simulink model "ofdm_transmitter"  (Simulink 8.5)
settings: Solver=ode45  StartTime=0.0  StopTime=inf  RelTol=1e-3
libraries: dspxfrm3 x2
settings Model: Creator=C4Josh  LastModifiedBy=C4Josh
settings DataIOCC: SignalLoggingSaveFormat=Dataset
settings OptimizationCC: BlockReduction=off  ConditionallyExecuteInputs=off  InlineParams=on  ExpressionDepthLimit=128
settings DebuggingCC: AlgebraicLoopMsg=error  UnderspecifiedInitializationDetection=Simplified  MergeDetectMultiDrivingBlocksExec=error  FcnCallInpInsideContextMsg=EnableAllAsError  StateNameClashWarn=none
settings HardwareCC: ProdHWDeviceType=ASIC/FPGA->ASIC/FPGA  ProdEqTarget=off
settings GRTTargetCC: CombineOutputUpdateFcns=on  GRTInterface=off
settings hdlcc: HDLCActiveTab=3

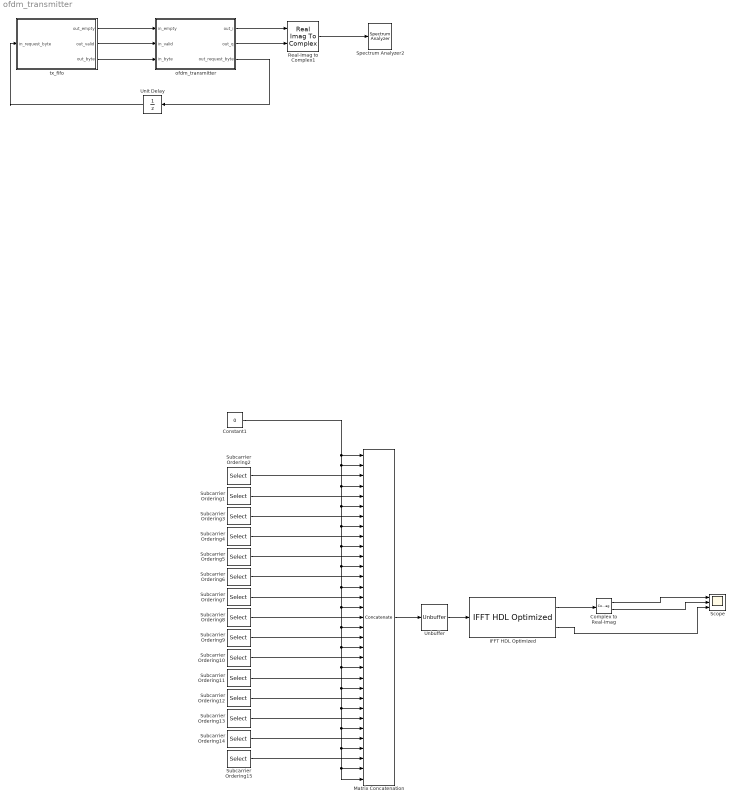
== system ofdm_transmitter ==
  Complex to Real-Imag : ComplexToRealImag
  Constant1 : Constant  Value=0  OutDataTypeStr=fixdt(1,12,7)
  IFFT HDL Optimized : dspxfrm3/IFFT HDL Optimized  BitReversedOutput=off  Normalize=on  FFTLengthSource=Property  FFTLength=64  RoundingMethod=Floor  OverflowAction=Saturate  ValidInputPort=off  ResetInputPort=off  StartOutputPort=off  EndOutputPort=off  SimulateUsing=Code generation
  Matrix Concatenation : Concatenate  NumInputs=33  Mode=Multidimensional array
  Real-Imag to Complex1 : RealImagToComplex
  Scope : Scope  NumInputPorts=3
      settings: YMin=-0.75~-0.75~1  YMax=1.5~0.75~1  SaveName=ScopeData2
  Spectrum Analyzer2 : SpectrumAnalyzer
  Subcarrier Ordering1 : Selector  InputPortWidth=45  Indices=4:6
  Subcarrier Ordering10 : Selector  InputPortWidth=45  Indices=28:30
  Subcarrier Ordering11 : Selector  InputPortWidth=45  Indices=31:33
  Subcarrier Ordering12 : Selector  InputPortWidth=45  Indices=34:36
  Subcarrier Ordering13 : Selector  InputPortWidth=45  Indices=37:39
  Subcarrier Ordering14 : Selector  InputPortWidth=45  Indices=40:42
  Subcarrier Ordering15 : Selector  InputPortWidth=45  Indices=40:42
  Subcarrier Ordering2 : Selector  InputPortWidth=45  Indices=1:3
  Subcarrier Ordering3 : Selector  InputPortWidth=45  Indices=7:9
  Subcarrier Ordering4 : Selector  InputPortWidth=45  Indices=10:12
  Subcarrier Ordering5 : Selector  InputPortWidth=45  Indices=13:15
  Subcarrier Ordering6 : Selector  InputPortWidth=45  Indices=16:18
  Subcarrier Ordering7 : Selector  InputPortWidth=45  Indices=19:21
  Subcarrier Ordering8 : Selector  InputPortWidth=45  Indices=22:24
  Subcarrier Ordering9 : Selector  InputPortWidth=45  Indices=25:27
  Unbuffer : Unbuffer  SampleBasedProcessing=Same as frame based
  Unit Delay : UnitDelay  SampleTime=-1
  ofdm_transmitter : Subsystem  TreatAsAtomicUnit=on
  tx_fifo : MATLAB Function  TreatAsAtomicUnit=on  SystemSampleTime=1/20e6
  wires:
  Subcarrier Ordering4/1 -> Matrix Concatenation/9
  Subcarrier Ordering11/1 -> Matrix Concatenation/23
  Subcarrier Ordering10/1 -> Matrix Concatenation/21
  Subcarrier Ordering8/1 -> Matrix Concatenation/17
  Subcarrier Ordering7/1 -> Matrix Concatenation/15
  Subcarrier Ordering3/1 -> Matrix Concatenation/7
  Subcarrier Ordering5/1 -> Matrix Concatenation/11
  Subcarrier Ordering15/1 -> Matrix Concatenation/31
  Subcarrier Ordering13/1 -> Matrix Concatenation/27
  Subcarrier Ordering9/1 -> Matrix Concatenation/19
  Subcarrier Ordering6/1 -> Matrix Concatenation/13
  IFFT HDL Optimized/1 -> Complex to Real-Imag/1
  IFFT HDL Optimized/2 -> Scope/3
  Constant1/1 -> Matrix Concatenation/2, Matrix Concatenation/4, Matrix Concatenation/6, Matrix Concatenation/8, Matrix Concatenation/10, Matrix Concatenation/14, Matrix Concatenation/16, Matrix Concatenation/20, Matrix Concatenation/24, Matrix Concatenation/26, Matrix Concatenation/32, Matrix Concatenation/33, Matrix Concatenation/30, Matrix Concatenation/28, Matrix Concatenation/22, Matrix Concatenation/18, Matrix Concatenation/12, Matrix Concatenation/1
  Complex to Real-Imag/1 -> Scope/1
  Complex to Real-Imag/2 -> Scope/2
  Subcarrier Ordering1/1 -> Matrix Concatenation/5
  Subcarrier Ordering14/1 -> Matrix Concatenation/29
  Subcarrier Ordering12/1 -> Matrix Concatenation/25
  Matrix Concatenation/1 -> Unbuffer/1
  Unbuffer/1 -> IFFT HDL Optimized/1
  Subcarrier Ordering2/1 -> Matrix Concatenation/3
  Real-Imag to Complex1/1 -> Spectrum Analyzer2/1
  tx_fifo/1(out_empty) -> ofdm_transmitter/1(in_empty)
  tx_fifo/2(out_valid) -> ofdm_transmitter/2(in_valid)
  tx_fifo/3(out_byte) -> ofdm_transmitter/3(in_byte)
  ofdm_transmitter/1(out_i) -> Real-Imag to Complex1/1
  ofdm_transmitter/2(out_q) -> Real-Imag to Complex1/2
  ofdm_transmitter/3(out_request_byte) -> Unit Delay/1
  Unit Delay/1 -> tx_fifo/1(in_request_byte)

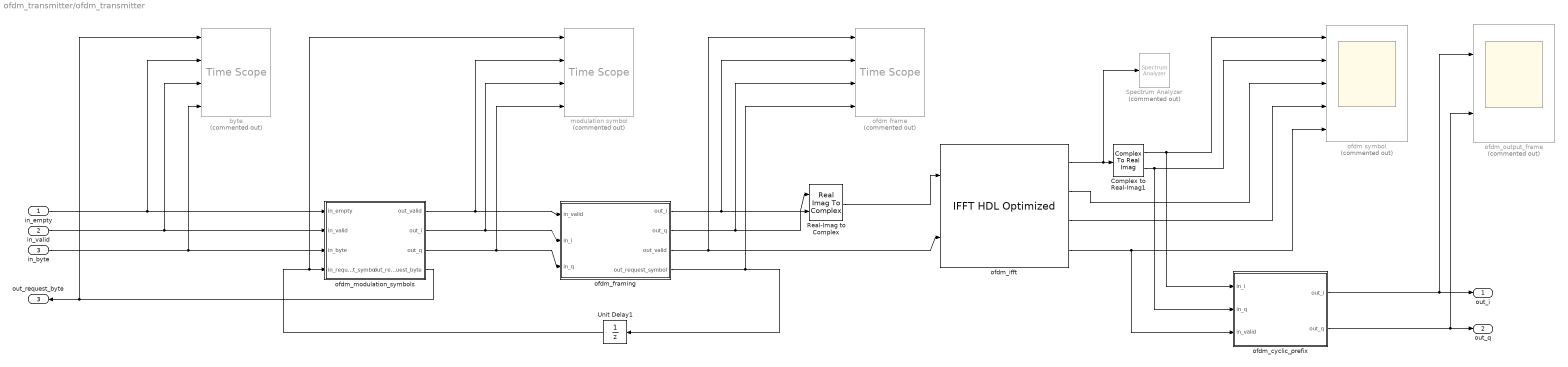
== system ofdm_transmitter/ofdm_transmitter ==
  in_empty : Inport
  in_valid : Inport  Port=2
  in_byte : Inport  Port=3
  " modulation symbol" : TimeScope  Commented=on  DefaultConfigurationName=spbscopes.TimeScopeBlockCfg  NumInputPorts=4
  Complex to Real-Imag1 : ComplexToRealImag
  Real-Imag to Complex : RealImagToComplex
  Spectrum Analyzer : SpectrumAnalyzer  Commented=on
  Unit Delay1 : UnitDelay  SampleTime=-1
  byte : TimeScope  Commented=on  DefaultConfigurationName=spbscopes.TimeScopeBlockCfg  NumInputPorts=4
  ofdm frame : TimeScope  Commented=on  DefaultConfigurationName=spbscopes.TimeScopeBlockCfg  NumInputPorts=4
  ofdm symbol : Scope  Commented=on  NumInputPorts=5
      settings: ShowLegends=on  YMin=-0.4~-0.75~0~0~0.95  YMax=0.4~0.75~1~1~1.05  SaveName=ScopeData3
  ofdm_cyclic_prefix : MATLAB Function  TreatAsAtomicUnit=on
  ofdm_framing : MATLAB Function  TreatAsAtomicUnit=on
  ofdm_ifft : dspxfrm3/IFFT HDL Optimized  BitReversedOutput=off  Normalize=on  FFTLengthSource=Property  FFTLength=64  RoundingMethod=Floor  OverflowAction=Saturate  ValidInputPort=on  ResetInputPort=off  StartOutputPort=on  EndOutputPort=on  SimulateUsing=Code generation
  ofdm_modulation_symbols : MATLAB Function  TreatAsAtomicUnit=on
  ofdm_output_frame : Scope  Commented=on  NumInputPorts=2
      settings: TickLabels=on  ShowLegends=on  TimeRange=800  YMin=-0.4~-0.7  YMax=0.35~0.7
  out_i : Outport
  out_q : Outport  Port=2
  out_request_byte : Outport  Port=3
  wires:
  in_empty/1 -> byte/2, ofdm_modulation_symbols/1(in_empty)
  in_valid/1 -> byte/3, ofdm_modulation_symbols/2(in_valid)
  in_byte/1 -> byte/4, ofdm_modulation_symbols/3(in_byte)
  ofdm_modulation_symbols/4(out_request_byte) -> out_request_byte/1, byte/1
  ofdm_modulation_symbols/1(out_valid) -> " modulation symbol"/2, ofdm_framing/1(in_valid)
  Unit Delay1/1 -> " modulation symbol"/1, ofdm_modulation_symbols/4(in_request_symbol)
  ofdm_modulation_symbols/2(out_i) -> " modulation symbol"/3, ofdm_framing/2(in_i)
  ofdm_modulation_symbols/3(out_q) -> " modulation symbol"/4, ofdm_framing/3(in_q)
  ofdm_framing/4(out_request_symbol) -> ofdm frame/4, Unit Delay1/1
  ofdm_framing/3(out_valid) -> ofdm frame/1, ofdm_ifft/2
  ofdm_framing/1(out_i) -> ofdm frame/2, Real-Imag to Complex/1
  ofdm_framing/2(out_q) -> ofdm frame/3, Real-Imag to Complex/2
  Real-Imag to Complex/1 -> ofdm_ifft/1
  ofdm_ifft/1 -> Complex to Real-Imag1/1, Spectrum Analyzer/1
  Complex to Real-Imag1/1 -> ofdm_cyclic_prefix/1(in_i), ofdm symbol/1
  Complex to Real-Imag1/2 -> ofdm_cyclic_prefix/2(in_q), ofdm symbol/2
  ofdm_ifft/2 -> ofdm symbol/3
  ofdm_ifft/3 -> ofdm symbol/4
  ofdm_ifft/4 -> ofdm_cyclic_prefix/3(in_valid), ofdm symbol/5
  ofdm_cyclic_prefix/2(out_q) -> ofdm_output_frame/2, out_q/1
  ofdm_cyclic_prefix/1(out_i) -> ofdm_output_frame/1, out_i/1

== matlab function ofdm_transmitter/ofdm_modulation_symbols ==
  data: out_valid output boolean size=1; out_i output fixdt(1,12,7) size=1; out_q output fixdt(1,12,7) size=1; in_empty input boolean size=1; in_valid input boolean size=1; out_request_byte output boolean size=1; in_byte input uint8 size=1; in_request_symbol input boolean size=1
function [out_valid, out_i, out_q, out_request_byte] = fcn(in_empty, in_valid, in_byte, in_request_symbol)
%#codegen

null = fi(0,1,12,7);

% MODULATION SYMBOL FORMAT
% 4-QAM, Grey coded, Minimum distance 2
%symbols = fi([-1+j -1-j 1+j 1-j],1,12,7);
symbols_i = fi([-1 -1 1 1],1,12,7);
symbols_q = fi([1 -1 1 -1],1,12,7);
bits_per_symbol = int8(2);
symbols_per_byte = 8/bits_per_symbol;
    
% by default, do nothing
out_request_byte = false;
out_i = null;
out_q = null;
out_valid = false;

% circular buffer for symbol storage
% the buffer length should evenly divide the number of symbols/byte
persistent buffer_i
if isempty(buffer_i)  
    buffer_i = repmat(null,1,2*symbols_per_byte);
end
persistent buffer_q
if isempty(buffer_q)  
    buffer_q = repmat(null,1,2*symbols_per_byte);
end
persistent read_index
if isempty(read_index)
    read_index = int8(0)
end
persistent write_index
if isempty(write_index)
    write_index = int8(0);
end

% we only receive valid input if we requested it
% if we have valid input, store the input
% this should *never* overflow
if in_valid
    
    % There are four symbols per byte
    % Map two bits to each symbol
    % This makes assumptions about the length of buffer
    % @review Is this the best way to do this?
    symbol1 = 1+bitand(bitshift(in_byte,-0),3);
    buffer_i(write_index+1) = symbols_i(symbol1);
    buffer_q(write_index+1) = symbols_q(symbol1);
    
    symbol2 = 1+bitand(bitshift(in_byte,-2),3);
    buffer_i(write_index+2) = symbols_i(symbol2);
    buffer_q(write_index+2) = symbols_q(symbol2);
    
    symbol3 = 1+bitand(bitshift(in_byte,-4),3);
    buffer_i(write_index+3) = symbols_i(symbol3);
    buffer_q(write_index+3) = symbols_q(symbol3);
    
    symbol4 = 1+bitand(bitshift(in_byte,-6),3);
    buffer_i(write_index+4) = symbols_i(symbol4);
    buffer_q(write_index+4) = symbols_q(symbol4);

    % we just wrote four symbols
    write_index = write_index + symbols_per_byte;
    if write_index >= length(buffer_i)
        write_index = int8(0);
    end
end

% determine how many symbols are buffered
buffered = int8(0);
if (read_index > write_index)
    buffered = (length(buffer_i) - read_index) + write_index;
elseif (read_index <= write_index)
    buffered = (write_index - read_index);
end

% if we have room for more symbols, request another byte
available = length(buffer_i) - buffered;
out_request_byte = (in_empty == 0) && (available >= symbols_per_byte);
%fprintf('[mod]read %d write %d request %d length %d buffered %d\n', ...
%    int8(read_index), int8(write_index), ...
%    int8(out_request_byte), int8(length(buffer_i)), int8(buffered));

% if there's buffered data, output a symbol
if in_request_symbol && (read_index ~= write_index)
    out_valid = true;
    out_i = buffer_i(read_index + 1);
    out_q = buffer_q(read_index + 1);
%    fprintf('[mod]read %d write %d symbol %d,%d\n', ...
%        int8(read_index), int8(write_index), ...
%        int8(out_i), int8(out_q));
    read_index = read_index + 1;
    if read_index >= length(buffer_i)
        read_index = int8(0);
    end
end

== matlab function tx_fifo ==
  data: out_empty output boolean size=1; out_valid output boolean size=1; in_request_byte input boolean size=1; out_byte output uint8 size=1
function [out_empty, out_valid, out_byte] = fcn(in_request_byte)
%#codegen

% assume we never empty
out_empty = false;

% we do not output by default
out_byte = uint8(0);
out_valid = false;

% fake data for our never empty source
persistent fake_data
if isempty(fake_data)
    fake_data = 3;
end

% if a byte is requested, supply a byte's worth of data
if in_request_byte
    out_byte = uint8(228);
    out_valid = true;
end

== matlab function ofdm_transmitter/ofdm_framing ==
  data: out_i output double; out_q output double; in_valid input double; in_i input double; in_q input double; out_valid output double; out_request_symbol output double
function [out_i, out_q, out_valid, out_request_symbol] = fcn(in_valid, in_i, in_q)
%#codegen

null = fi(0,1,12,7);
frame_size = int8(64);
% the number of symbols grouped in contiguous subcarries
symbols_per_run = 3;
% pilots are inserted between symbol runs
pilots_i = fi([1 0 -1 0],1,12,7);
pilots_q = fi([0 1 0 -1],1,12,7);

% this creates a frame that looks like:
% [ null null (pilot run)+ null ]
% given the current parameters, that means
% 16 pilots / ofdm frame
% 3xnull / ofdm frame
% 45 modulation symbols / ofdm frame
% 2 bits / modulation symbol
% 90 bits / ofdm frame

% default behavior
out_request_symbol = false;
out_valid = false;
out_i = null;
out_q = null;

% circular buffer for symbol storage
persistent buffer_i
if isempty(buffer_i)  
    buffer_i = repmat(null,1,frame_size);
end
persistent buffer_q
if isempty(buffer_q)  
    buffer_q = repmat(null,1,frame_size);
end
persistent read_index
if isempty(read_index)
    read_index = int8(0);
end
persistent write_index
if isempty(write_index)
    write_index = int8(0);
end

% framing state
persistent frame_index
persistent pilot_index
if isempty(pilot_index)
    pilot_index = int8(1);
end
persistent symbol_count
if isempty(symbol_count)
    symbol_count = int8(0);
end

% is this the first symbol in a frame?
frame_begin = (write_index == 0);
% is this the last symbol in a run?
run_end = (symbol_count == (symbols_per_run - 1));
% is this the last write in the frame?
% the frame will end with a (symbol)(pilot)(null)
frame_end = ((write_index + 2) == (frame_size - 1));
%fprintf('[frm]valid %d %f,%f write %d frame begin %d end %d run %d end %d\n', ...
%    int8(in_valid), double(in_i), double(in_q), ...
%    int8(write_index), ...
%    int8(frame_begin), int8(frame_end), ...
%    int8(symbol_count), int8(run_end));

% The following scenarios can occur:
% (null)(null)(pilot)(symbol)
% (symbol)(pilot)(null)
% (symbol)(pilot)
% (symbol)
if in_valid
    if frame_begin
        % (null)(null)(pilot)(symbol)
%        fprintf('[frm]write %d nullx2 pilot %d %d,%d symbol %d %d,%d\n', ...
%            int8(write_index), ...
%            int8(pilot_index), int8(pilots_i(pilot_index)), int8(pilots_q(pilot_index)), ...
%            int8(symbol_count), int8(in_i), int8(in_q));
        buffer_i(write_index+1) = null;
        buffer_q(write_index+1) = null;
        buffer_i(write_index+2) = null;
        buffer_q(write_index+2) = null;
        buffer_i(write_index+3) = pilots_i(1);
        buffer_q(write_index+3) = pilots_q(1);
        buffer_i(write_index+4) = in_i;
        buffer_q(write_index+4) = in_q;
        write_index = int8(4);
        symbol_count = int8(1);
        pilot_index = int8(2);
    elseif frame_end
        % (symbol)(pilot)(null)
%        fprintf('[frm]write %d symbol %d %d,%d pilot %d %d,%d null\n', ...
%            int8(write_index), ...
%            int8(symbol_count), int8(in_i), int8(in_q), ...
%            int8(pilot_index), int8(pilots_i(pilot_index)), int8(pilots_q(pilot_index)));
        buffer_i(write_index+1) = in_i;
        buffer_q(write_index+1) = in_q;
        buffer_i(write_index+2) = pilots_i(pilot_index);
        buffer_q(write_index+2) = pilots_q(pilot_index);
        buffer_i(write_index+3) = null;
        buffer_q(write_index+3) = null;
        write_index = int8(0);
        symbol_count = int8(0);
        pilot_index = int8(1);
    elseif run_end
        % (symbol)(pilot)
%        fprintf('[frm]write %d symbol %d %d,%d pilot %d %d,%d\n', ...
%            int8(write_index), ...
%            int8(symbol_count), int8(in_i), int8(in_q), ...
%            int8(pilot_index), int8(pilots_i(pilot_index)), int8(pilots_q(pilot_index)));
        buffer_i(write_index+1) = in_i;
        buffer_q(write_index+1) = in_q;
        buffer_i(write_index+2) = pilots_i(pilot_index);
        buffer_q(write_index+2) = pilots_q(pilot_index);
        write_index = write_index + 2;
        symbol_count = int8(0);
        pilot_index = pilot_index + 1;
        if pilot_index == length(pilots_i)
            pilot_index = int8(1);
        end
    else
        % (symbol)
%        fprintf('[frm]write %d symbol %d %d,%d\n', ...
%            int8(write_index), ...
%            int8(symbol_count), int8(in_i), int8(in_q));
        buffer_i(write_index+1) = in_i;
        buffer_q(write_index+1) = in_q;
        write_index = write_index + 1;
        symbol_count = symbol_count + 1;
    end
end

% determine how many symbols are buffered
buffered = int8(0);
if (read_index > write_index)
    buffered = (length(buffer_i) - read_index) + write_index;
elseif (read_index <= write_index)
    buffered = (write_index - read_index);
end

% we can write at *most* a 2xnull, a pilot, and a symbol
% if there's room enough to support as much, reques t a symbol
available = length(buffer_i) - buffered;
out_request_symbol = (available >= 4);

% output i/q if there's something buffered
if read_index ~= write_index
    out_valid = true;
    out_i = buffer_i(read_index + 1);
    out_q = buffer_q(read_index + 1);
    read_index = read_index + 1;
    if read_index >= length(buffer_i)
        read_index = int8(0);
    end
end

== matlab function ofdm_transmitter/ofdm_cyclic_prefix ==
  data: out_i output fixdt(1,12,7) size=1; out_q output fixdt(1,12,7) size=1; in_i input fixdt(1,12,7) size=1; in_q input fixdt(1,12,7) size=1; in_valid input boolean size=1
function [out_i, out_q]  = fcn(in_i, in_q, in_valid)
%#codegen

% constants
% ifft_size = 64;
% cyclic_prefix = 16;
null = fi(0,1,12,7);

% persistent state
persistent buffer_i
if isempty(buffer_i)  
    buffer_i = repmat(null,1,80);
end
persistent buffer_q
if isempty(buffer_q)  
    buffer_q = repmat(null,1,80);
end
persistent read_index
if isempty(read_index)
    read_index = int8(0);
end
persistent write_index
if isempty(write_index)
    write_index = int8(16);
end

% default behavior
out_i = null;
out_q = null;

% determine how many samples are buffered
buffered = int8(0);
if (read_index > write_index)
    buffered = (length(buffer_i) - read_index) + write_index;
elseif (read_index <= write_index)
    buffered = (write_index - read_index);
end

% if there's more than a cyclic prefix worth of space available,
% request input
available = length(buffer_i) - buffered;

% if the input is valid and there's space available, store the input
if in_valid && (available > 0)
%    fprintf('[cp]write %d symbol %f,%f\n', ...
%        int8(write_index), double(in_i), double(in_q));
    buffer_i(write_index + 1) = in_i;
    buffer_q(write_index + 1) = in_q;
    write_index = write_index + 1;
    if write_index >= length(buffer_i)
        write_index = int8(16);
    end
end

% if there are samples buffered, output
if read_index ~= write_index
    out_i = buffer_i(read_index + 1);
    out_q = buffer_q(read_index + 1);
%    fprintf('[cp]read %d symbol %f,%f\n', ...
%        int8(read_index), double(out_i), double(out_q));
    read_index = read_index + 1;
    if read_index >= length(buffer_i)
        read_index = int8(0);
    end
end
